simulink model "TestCinematiqueNew"  (R2024b)
settings: Solver=ode45  StartTime=0.0  StopTime=10.0  RelTol=1e-3  EnableMultiTasking=on
undefined symbols (not defined in the file): EngineSpeedTest, EngineSpeedTimeTest
settings Model: Creator=a030141  LastModifiedBy=ramse
settings SolverCC: AlgebraicLoopSolver=TrustRegion
settings DataIOCC: LimitDataPoints=on  SaveFormat=Array  SignalLoggingSaveFormat=ModelDataLogs  ReturnWorkspaceOutputs=off  SignalLoggingName=sigsOut
settings OptimizationCC: InitFltsAndDblsToZero=on  LifeSpan=inf
settings DebuggingCC: SaveWithParameterizedLinksMsg=none  UnderspecifiedInitializationDetection=Classic  MergeDetectMultiDrivingBlocksExec=none  SignalResolutionControl=TryResolveAllWithWarning  MultiTaskDSMMsg=warning  MultiTaskCondExecSysMsg=none  FcnCallInpInsideContextMsg=warning  UnconnectedInputMsg=warning  UnconnectedOutputMsg=warning  UnconnectedLineMsg=warning  SFUnexpectedBacktrackingDiag=warning  SFNoUnconditionalDefaultTransitionDiag=warning  SFExecutionAtInitializationDiag=none  ArithmeticOperatorsInVariantConditions=warning
settings HardwareCC: ProdBitPerPointer=32  ProdBitPerSizeT=32  ProdBitPerPtrDiffT=32  ProdLargestAtomicFloat=None  ProdIntDivRoundTo=Undefined  ProdEndianess=Unspecified  ProdWordSize=32  ProdHWDeviceType=32-bit Generic  TargetUnknown=on
settings ModelReferenceCC: PropagateSignalLabelsOutOfModel=off
settings RTWCC: GPUComputeCapability=3.5
settings CodeAppCC: StateflowObjectComments=on
settings GRTTargetCC: TargetFcnLib=ansi_tfl_tmw.mat  TargetLangStandard=C89/C90 (ANSI)  CombineOutputUpdateFcns=off  GRTInterface=on
settings ConfigComp: CovMetricSettings=dw  CovSaveCumulativeToWorkspaceVar=on  CovSaveSingleToWorkspaceVar=on

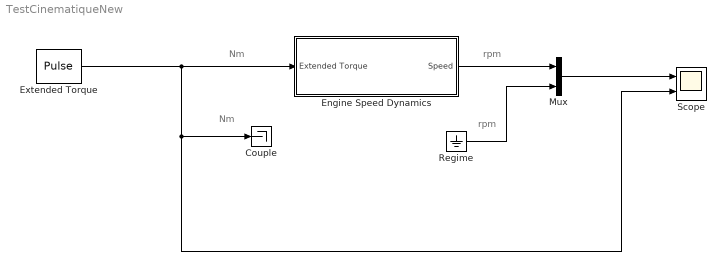
== system TestCinematiqueNew ==
  note: rpm
  note: rpm
  note: Nm
  note: Nm
  Couple : Terminator
  Engine Speed Dynamics : Subsystem
  Extended Torque : DiscretePulseGenerator  PulseType=Time based  PulseWidth=50
  Mux : Mux  Inputs=2
  Regime : Ground
  Scope : Scope  NumInputPorts=2
  wires:
  Extended Torque/1 -> Engine Speed Dynamics/1(Extended Torque), Scope/2, Couple/1
  Engine Speed Dynamics/1(Speed) -> Mux/1
  Mux/1 -> Scope/1
  Regime/1 -> Mux/2

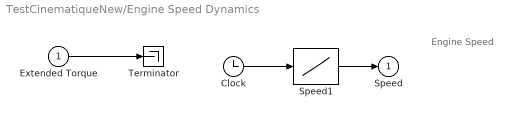
== system TestCinematiqueNew/Engine Speed Dynamics ==
  note: Engine Speed
  Extended Torque : Inport
  Clock : Clock
  Speed1 : Lookup  InputValues=EngineSpeedTimeTest  Table=EngineSpeedTest
  Terminator : Terminator
  Speed : Outport
  wires:
  Speed1/1 -> Speed/1
  Clock/1 -> Speed1/1
  Extended Torque/1 -> Terminator/1
